simulink model "c_hdd"  (Simulink 6.3)
settings: Solver=ode23tb  StartTime=0.0  StopTime=0.004  RelTol=1e-3
values from neighbouring files (symbols this model uses):
  b1 = 0.006    [init_c_hdd.m]    (also in init_d_hdd.m; mod_hdd.m)
  b2 = 0    [init_c_hdd.m]    (also in init_d_hdd.m; mod_hdd.m)
  b3 = 0.013    [init_c_hdd.m]    (also in init_d_hdd.m; mod_hdd.m)
  b4 = -0.0018    [init_c_hdd.m]    (also in init_d_hdd.m; mod_hdd.m)
  b5 = 0.723    [init_c_hdd.m]    (also in init_d_hdd.m; mod_hdd.m)
  b6 = -0.0015    [init_c_hdd.m]    (also in init_d_hdd.m; mod_hdd.m)
  b7 = 0.235    [init_c_hdd.m]    (also in init_d_hdd.m; mod_hdd.m)
  b8 = -0.0263    [init_c_hdd.m]    (also in init_d_hdd.m; mod_hdd.m)
  emax = 12    [init_c_hdd.m]    (also in init_d_hdd.m; lsh_hdd.m = info.emax)
  J = 6.3857*10^(-6)    (= 6.3857e-06)    [init_c_hdd.m]    (also in init_d_hdd.m; mod_hdd.m = ureal('J',6.3857*10^(-6),'Percentage',10))
  Kb = 9.183*10^(-2)    (= 0.09183)    [init_c_hdd.m]    (also in init_d_hdd.m; mod_hdd.m)
  kf = 0.0006    [init_c_hdd.m]    (also in init_d_hdd.m)
  Kpa = 10    [init_c_hdd.m]    (also in init_d_hdd.m; mod_hdd.m)
  Kt = 9.183*10^(-2)    (= 0.09183)    [init_c_hdd.m]    (also in init_d_hdd.m; mod_hdd.m = ureal('Kt',9.183*10^(-2),'Percentage',10))
  Ky = 1.2    [init_c_hdd.m]    (also in init_d_hdd.m; mod_hdd.m = ureal('Ky',1.2,'Percentage',5))
  R = 5.08*10^(-2)    (= 0.0508)    [init_c_hdd.m]    (also in init_d_hdd.m; mod_hdd.m)
  Rc = Rcoil + Rs    (= 8.2)    [init_c_hdd.m]    (also in init_d_hdd.m; mod_hdd.m)
  Rs = 0.2    [init_c_hdd.m]    (also in init_d_hdd.m; mod_hdd.m)
  tau = Lcoil/Rc    (= 0.000121951219512)    [init_c_hdd.m]    (also in init_d_hdd.m; mod_hdd.m)
  Tf1 = 0.1    [init_c_hdd.m]    (also in init_d_hdd.m)
  Tf2 = 0.001    [init_c_hdd.m]    (also in init_d_hdd.m)
  tpm = 10^6    (= 1000000)    [init_c_hdd.m]    (also in init_d_hdd.m; mod_hdd.m)
  w1 = 2*pi*50    (= 314.159265359)    [init_c_hdd.m]    (also in init_d_hdd.m; mod_hdd.m = ureal('w1',2*pi*50,'Percentage',5))
  w2 = 2*pi*2200    (= 13823.0076758)    [init_c_hdd.m]    (also in init_d_hdd.m; mod_hdd.m = ureal('w2',2*pi*2200,'Percentage',12))
  w3 = 2*pi*6400    (= 40212.3859659)    [init_c_hdd.m]    (also in init_d_hdd.m; mod_hdd.m = ureal('w3',2*pi*6400,'Percentage',8))
  w4 = 2*pi*8800    (= 55292.0307032)    [init_c_hdd.m]    (also in init_d_hdd.m; mod_hdd.m = ureal('w4',2*pi*8800,'Percentage',15))
  z1 = 0.3    [init_c_hdd.m]    (also in init_d_hdd.m; mod_hdd.m = ureal('z1',0.3,'Percentage',5))
  z2 = 0.024    [init_c_hdd.m]    (also in init_d_hdd.m; mod_hdd.m = ureal('z2',0.024,'Percentage',8))
  z3 = 0.129    [init_c_hdd.m]    (also in init_d_hdd.m; mod_hdd.m = ureal('z3',0.129,'Percentage',10))
  z4 = 0.173    [init_c_hdd.m]    (also in init_d_hdd.m; mod_hdd.m = ureal('z4',0.173,'Percentage',10))
undefined symbols (not defined in the file or in its folder): ak, bk, ck, dk
libraries: simulink x1
settings Model: LastModifiedBy=Petko Petkov  StrictBusMsg=None
settings DataIOCC: SignalLoggingName=sigsOut
settings OptimizationCC: BlockReduction=off  BooleanDataType=off  InlineInvariantSignals=on
settings DebuggingCC: SolverPrmCheckMsg=none
settings HardwareCC: TargetUnknown=on
settings GRTTargetCC: ModelReferenceCompliant=off  MatFileLogging=off

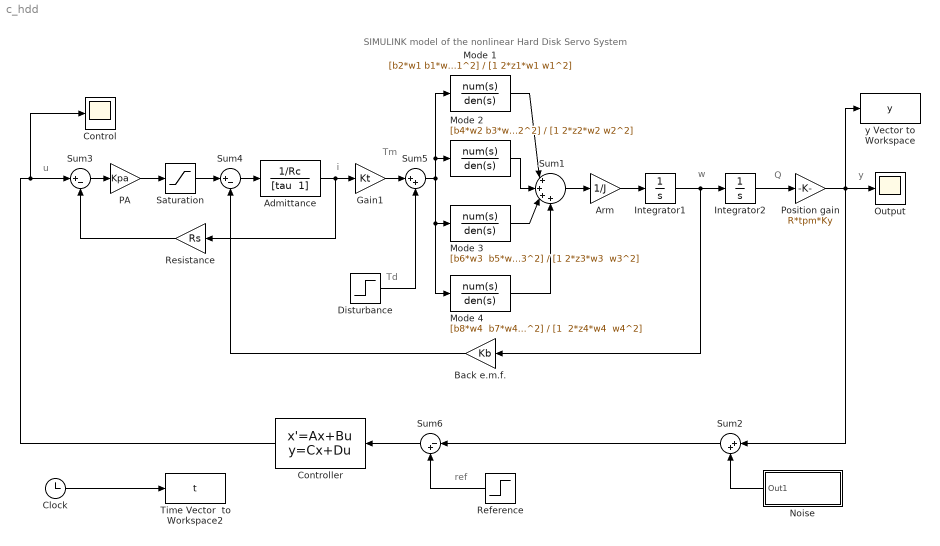
== system c_hdd ==
  note: ref
  note: i
  note: Td
  note: u
  note: Tm
  note: SIMULINK model of the nonlinear Hard Disk Servo System
  note: w
  note: y
  note: Q
  Admittance : TransferFcn  Numerator=1/Rc  Denominator="[tau  1]"
  Arm : Gain  Gain=1/J  SaturateOnIntegerOverflow=on
  Back e.m.f. : Gain  Orientation=left  Gain=Kb  SaturateOnIntegerOverflow=on
  Clock : Clock
  Control : Scope
      settings: TimeRange=0.01  YMin=5500  YMax=11000
  Controller : StateSpace  Orientation=left  A=ak  B=bk  C=ck  D=dk
  Disturbance : Step  Time=0  After=0  SampleTime=0
  Gain1 : Gain  Gain=Kt  SaturateOnIntegerOverflow=on
  Integrator1 : Integrator
  Integrator2 : Integrator
  Mode 1 : TransferFcn  Numerator=[b2*w1 b1*w1^2]  Denominator=[1 2*z1*w1 w1^2]
  Mode 2 : TransferFcn  Numerator=[b4*w2 b3*w2^2]  Denominator=[1 2*z2*w2 w2^2]
  Mode 3 : TransferFcn  Numerator="[b6*w3  b5*w3^2]"  Denominator="[1 2*z3*w3  w3^2]"
  Mode 4 : TransferFcn  Numerator="[b8*w4  b7*w4^2]"  Denominator="[1  2*z4*w4  w4^2]"
  Noise : Subsystem  Orientation=left
  Output : Scope
      settings: TimeRange=0.01  YMin=0  YMax=0.25
  PA : Gain  Gain=Kpa  SaturateOnIntegerOverflow=on
  Position gain : Gain  Gain=R*tpm*Ky  SaturateOnIntegerOverflow=on
  Reference : Step  Orientation=left  Time=0  After=1.2  SampleTime=0
  Resistance : Gain  Orientation=left  Gain=Rs  SaturateOnIntegerOverflow=on
  Saturation : Saturate  UpperLimit=emax  LowerLimit=-emax
  Sum1 : Sum  Inputs=|++++  SaturateOnIntegerOverflow=on  InputSameDT=on
  Sum2 : Sum  Orientation=left  Inputs=|++  SaturateOnIntegerOverflow=on  InputSameDT=on
  Sum3 : Sum  Inputs=|+-  SaturateOnIntegerOverflow=on  InputSameDT=on
  Sum4 : Sum  Inputs=|+-  SaturateOnIntegerOverflow=on  InputSameDT=on
  Sum5 : Sum  Inputs=|++  SaturateOnIntegerOverflow=on  InputSameDT=on
  Sum6 : Sum  Orientation=left  Inputs=|-+  SaturateOnIntegerOverflow=on  InputSameDT=on
  Time Vector  to Workspace2 : ToWorkspace  VariableName=t  SampleTime=-1  SaveFormat=Array
  y Vector to Workspace : ToWorkspace  VariableName=y  SampleTime=-1  SaveFormat=Array
  wires:
  Mode 1/1 -> Sum1/1
  Mode 2/1 -> Sum1/2
  Mode 4/1 -> Sum1/4
  PA/1 -> Saturation/1
  Resistance/1 -> Sum3/2
  Sum3/1 -> PA/1
  Back e.m.f./1 -> Sum4/2
  Mode 3/1 -> Sum1/3
  Sum4/1 -> Admittance/1
  Admittance/1 -> Resistance/1, Gain1/1
  Sum5/1 -> Mode 2/1, Mode 1/1, Mode 3/1, Mode 4/1
  Disturbance/1 -> Sum5/2
  Gain1/1 -> Sum5/1
  Controller/1 -> Sum3/1, Control/1
  Clock/1 -> Time Vector  to Workspace2/1
  Noise/1(Out1) -> Sum2/2
  Reference/1 -> Sum6/2
  Sum2/1 -> Sum6/1
  Integrator1/1 -> Back e.m.f./1, Integrator2/1
  Position gain/1 -> y Vector to Workspace/1, Sum2/1, Output/1
  Arm/1 -> Integrator1/1
  Integrator2/1 -> Position gain/1
  Sum6/1 -> Controller/1
  Sum1/1 -> Arm/1
  Saturation/1 -> Sum4/1

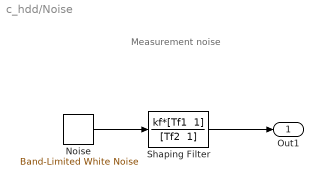
== system c_hdd/Noise ==
  note: Measurement noise
  Noise : simulink/Sources/Band-Limited White Noise  Cov=10^(-4)  Ts=0.1  seed=[23341]
  Shaping Filter : TransferFcn  Numerator="kf*[Tf1  1]"  Denominator="[Tf2  1]"
  Out1 : Outport
  wires:
  Noise/1 -> Shaping Filter/1
  Shaping Filter/1 -> Out1/1
